simulink model "untitled"  (Simulink 9.2)
settings: Solver=ode45  StartTime=0.0  StopTime=50.0  MaxStep=0.1  RelTol=1e-3
libraries: simulink_extras x1
settings Model: Creator=Alumno  LastModifiedBy=Alumno
settings DataIOCC: LimitDataPoints=off  SaveFormat=Dataset  SignalLoggingSaveFormat=Dataset
settings OptimizationCC: LifeSpan=auto
settings DebuggingCC: UnderspecifiedInitializationDetection=Simplified  MergeDetectMultiDrivingBlocksExec=error  FcnCallInpInsideContextMsg=error  StateNameClashWarn=none  SFUnexpectedBacktrackingDiag=error  SFNoUnconditionalDefaultTransitionDiag=error  SFExecutionAtInitializationDiag=warning
settings HardwareCC: ProdBitPerPointer=64  ProdBitPerSizeT=64  ProdBitPerPtrDiffT=64  ProdLargestAtomicFloat=Float  ProdIntDivRoundTo=Zero  ProdEndianess=LittleEndian  ProdWordSize=64  ProdHWDeviceType=Intel->x86-64 (Windows64)
settings ModelReferenceCC: PropagateSignalLabelsOutOfModel=on
settings SFSimCC: SimUseLocalCustomCode=on
settings RTWCC: RTWUseLocalCustomCode=on
settings CodeAppCC: StateflowObjectComments=off
settings GRTTargetCC: TargetLangStandard=C99 (ISO)  GeneratePreprocessorConditionals=Use local settings  CombineOutputUpdateFcns=on  GRTInterface=off
settings ConfigComp: CovMetricSettings=dwe  CovHtmlReporting=off  CovSaveCumulativeToWorkspaceVar=off  CovSaveSingleToWorkspaceVar=off  CovExternalEMLEnable=on

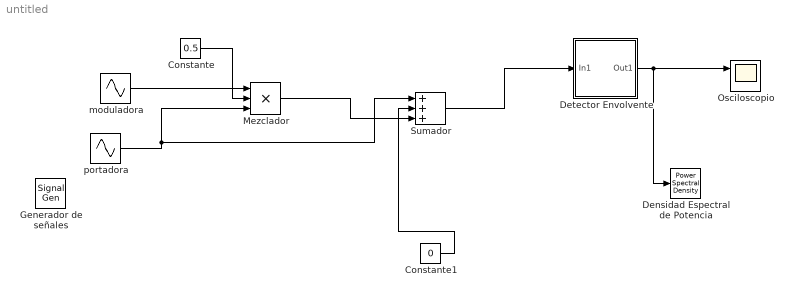
== system untitled ==
  Constante : Constant  Value=0.5
  Constante1 : Constant  Value=0
  Densidad Espectral de Potencia : simulink_extras/Additional Sinks/Power Spectral Density  npts=512  fftpts=512  HowOften=64  sampleT=0.1
      settings: SourceProductName=Simulink  SourceProductBaseCode=SL
  Detector Envolvente : Subsystem  mask(Envelope Detector (TELECO UPCT)){Tau=0.5}
      mask prompts: Tau "Tau (R*C) [sg]"
      mask help:
      | The Envelope Detector allows the demodulation of amplitude modulated signal which are not overmodulated.
      |
      | Select Tau (R*C) [s] with a value much higher than Tp (Carrier Period) and lower than Tm (Modulating Signal Period).
      |
      | E.g. If Tp=0.001 s, and Tm=10 s, then a suitable Tau could be between 0.1 and 1 s.
      mask Display: plot([0 0.0100 0.020 0.0301 0.0402 0.0502 0.06030 0.07035 0.08040 0.0904 0.1005 0.11055 0.1206 0.1306532 0.1407 0.15075 0.160804 0.17085 0.1809045 0.19095 0.2010 0.211055 0.2211 0.231155 0.24120 0.251256 0.26130 0.27135 0.28140703 0.291457 0.301507 0.3115 0.321608 0.331658 0.34170 0.35175 0.361809 0.371859 0.38190 0.39195 0.40201 0.412 0.422110552763819 0.432160804020101 0.442211055276382 0.452261306532663 0.462311557788945 0.472361809045226 0.482412060301508 0.492462311557789],[1.50000000000000 1.35725612705394 1.22809612961697 1.11122733102258 1.21161108958560 1.47509990887487 1.33472559289142 1.20770965925839 1.09278088982045 1.17321137879314 1.40287899306847 1.26937740590496 1.14858017447223 1.03927831947674 1.09864678512587 1.29052485666534 1.16771517921629 1.05659238776346 0.956044328060342 0.995576679540851 1.14920747660210 1.03984592591626 0.940891502761281 0.851353838010491 0.874697418425945 0.992951895818910 0.898460029646694 0.812960253434026 0.735596856683103 0.748707875672720 0.837224292404762 0.75755 0.68546 0.62023 0.63104 0.6973 0.6310 0.57096 0.51662 0.5345 0.5870 0.5312 0.48067 0.4349 0.4700 0.5170 0.4678 0.4233 0.3830 0.4454],[0 0.0100502512562814 0.0201005025125628 0.0301507537688442 0.0402010050251256 0.0502512562814070 0.0603015075376884 0.0703517587939699 0.0804020100502513 0.0904522613065327 0.100502512562814 0.110552763819095 0.120603015075377 0.130653266331658 0.140703517587940 0.150753768844221 0.160804020100503 0.170854271356784 0.180904522613065 0.190954773869347 0.201005025125628 0.211055276381910 0.221105527638191 0.231155778894472 0.241206030150754 0.251256281407035 0.261306532663317 0.271356783919598 0.281407035175879 0.291457286432161 0.301507537688442 0.311557788944724 0.321608040201005 0.331658291457286 0.341708542713568 0.351758793969849 0.361809045226131 0.371859296482412 0.381909547738693 0.391959798994975 0.402010050251256 0.412060301507538 0.422110552763819 0.432160804020101 0.442211055276382 0.452261306532663 0.462311557788945 0.472361809045226 0.482412060301508 0.492462311557789], [1.50000000000000 1.20993126439682 0.453301106657544 -0.474172583029756 -1.21161108958560 -1.47509990887487 -1.16831719880494 -0.418047916584565 0.478613777302988 1.17321137879314 1.40287899306847 1.09087247839569 0.371835504257245 -0.466298299188217 -1.09864678512587 -1.29052485666534 -0.985159188934220 -0.318978844871803 0.438787868134165 0.995576679540851 1.14920747660210 0.861359170684520 0.264132949337291 -0.399486171411829 -0.874697418425945 -0.992951895818910 -0.731189040830292 -0.211736977904714 0.353374570524558 0.748707875672720 0.837224292404762 0.606685035222284 0.165519860648553 -0.306548903245726 -0.631049231141791 -0.697375278761685 -0.498984597632528 -0.128122278411314 0.265600709413535 0.534545276542671 0.587098567823176 0.417229181498486 0.100873701918498 -0.236906206282143 -0.470081999110723 -0.517061222036970 -0.367697445635419 -0.0837430370887885 0.225899803116156 0.445463423116636])
  Generador de señales : SignalGenerator  Frequency=10  Units=rad/sec
  Mezclador : Product  Inputs=3  SaturateOnIntegerOverflow=on  RndMeth=Zero  InputSameDT=on  OutDataTypeStr=Inherit: Same as first input
  Osciloscopio : Scope  NumInputPorts=2
  "Sumador " : Sum  Inputs=+++  SaturateOnIntegerOverflow=on  InputSameDT=on  OutDataTypeStr=Inherit: Same as first input
  "moduladora " : Sin  SampleTime=0
  "portadora " : Sin  Amplitude=10  Frequency=10  SampleTime=0
  wires:
  "moduladora "/1 -> Mezclador/1
  "portadora "/1 -> "Sumador "/1, Mezclador/3
  Mezclador/1 -> "Sumador "/3
  Constante/1 -> Mezclador/2
  "Sumador "/1 -> Detector Envolvente/1(In1)
  Detector Envolvente/1(Out1) -> Osciloscopio/1, Densidad Espectral de Potencia/1
  Constante1/1 -> "Sumador "/2

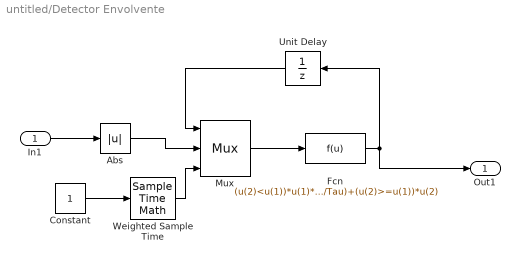
== system untitled/Detector Envolvente ==
  In1 : Inport
  Abs : Abs
  Constant : Constant
  Fcn : Fcn  Expr=(u(2)<u(1))*u(1)*exp(-u(3)/Tau)+(u(2)>=u(1))*u(2)
  Mux : Mux  Inputs=3
      settings: DisplayOption=signals
  Unit Delay : UnitDelay  SampleTime=-1
  Weighted Sample Time : SampleTimeMath  TsampMathOp=Ts Only
  Out1 : Outport
  wires:
  Weighted Sample Time/1 -> Mux/3
  Constant/1 -> Weighted Sample Time/1
  In1/1 -> Abs/1
  Fcn/1 -> Unit Delay/1, Out1/1
  Abs/1 -> Mux/2
  Mux/1 -> Fcn/1
  Unit Delay/1 -> Mux/1
